simulink model "MLIB_VMac_BAM_FLT"  (Simulink 8.3)
settings: Solver=ode45  StartTime=0.0  StopTime=10.0  RelTol=1e-3
settings Model: Creator=RE004C  LastModifiedBy=B17364
settings OptimizationCC: ExpressionDepthLimit=2147483647
settings DebuggingCC: FcnCallInpInsideContextMsg=UseLocalSettings  StrictBusMsg=Warning
settings HardwareCC: ProdLargestAtomicInteger=Long  ProdLargestAtomicFloat=Double  ProdIntDivRoundTo=Zero  ProdEndianess=BigEndian  ProdHWDeviceType=Freescale->32-bit PowerPC

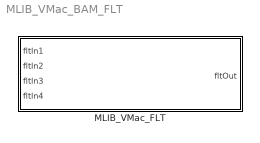
== system MLIB_VMac_BAM_FLT ==
  MLIB_VMac_FLT : Subsystem  mask(MLIB_VMac_FLT){}
      mask help: Bit accurate model of vector multiply accumulate function. All parameters as well as input and output are 32-bit integers.
      mask init:
      | pos = get_param(gcb, 'Position');width = pos(3) - pos(1); height = pos(4) - pos(2);tX=width/2;tY=height*0.9;
      mask Display: color('black');port_label('input',1,'fltIn1');port_label('input',2,'fltIn2');port_label('input',3,'fltIn3');port_label('input',4,'fltIn4');port_label('output',1,'fltOut');color('black');disp('MLIB_VMac_FLT');color('blue');text(tX,tY, 'BAM', 'horizontalAlignment', 'center');

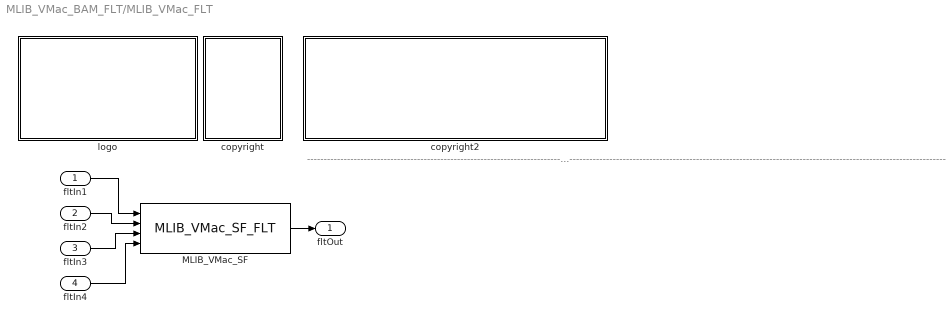
== system MLIB_VMac_BAM_FLT/MLIB_VMac_FLT ==
  note: ---------------------------------------------------------------------------------------------------------------------------------------------------------------------------------------------------
  fltIn1 : Inport
  fltIn2 : Inport  Port=2
  fltIn3 : Inport  Port=3
  fltIn4 : Inport  Port=4
  MLIB_VMac_SF : S-Function  FunctionName=MLIB_VMac_SF_FLT  EnableBusSupport=off
  copyright : Subsystem
      mask Display:
      | text(10,90,'FILE:');text(10,75,'DESRIPTION:')
      | text(10,60,'COPYRIGHT:')
      | text(10,45,'VERSION:')
      | text(10,30,'DATE:')
  copyright2 : Subsystem
      mask Display:
      | text(10,90,'MLIB_VMac_BAM_FLT.mdl');text(10,75,'Vector multiply accumulate.');text(10,60,'Freescale')
      | text(10,45,'0.1');text(10,30,'25-Aug-2011');
  logo : Subsystem
      mask Display: image(imread('logo.jpg'))
  fltOut : Outport
  wires:
  fltIn1/1 -> MLIB_VMac_SF/1
  fltIn2/1 -> MLIB_VMac_SF/2
  fltIn3/1 -> MLIB_VMac_SF/3
  fltIn4/1 -> MLIB_VMac_SF/4
  MLIB_VMac_SF/1 -> fltOut/1

== system MLIB_VMac_BAM_FLT/MLIB_VMac_FLT/copyright ==

== system MLIB_VMac_BAM_FLT/MLIB_VMac_FLT/copyright2 ==

== system MLIB_VMac_BAM_FLT/MLIB_VMac_FLT/logo ==
